simulink model "heatlib_demo"  (R2014b)
settings: Solver=ode1  StartTime=t(1)  StopTime=t(end)  FixedStep=ts  RelTol=1e-3
InitFcn:
  | % Copyright (C) 2014 Kai Kruppa
  | %
  | % This program is free software: you can redistribute it and/or modify it under
  | % the terms of the GNU General Public License as published by the Free Software
  | % Foundation, either version 3 of the License, or (at your option) any later version.
  | %
  | % This program is distributed in the hope that it will be useful, but WITHOUT ANY
  | % WARRANTY; without even the implied warranty of MERCHANTABILITY or
  | % FITNESS FOR A PARTICULAR PURPOSE. See the GNU General Public License for
  | % more details.
  | %
  | % You should have received a copy of the GNU General Public License along with
  | % this program.  If not, see <http://www.gnu.org/licenses/>.
  | 
  | % Kompiliere CMEX-Funktion falls notwendig
  | if exist('storage_tank','file') ~= 3
  |     mex storage_tank.c;
  | end
  | 
  | % Simulationseingang für Modell
  | ts     = 1;
  | N      = 24*60;
  | t      = 60*(0:N-1)';
  | an_aus_BHKW  = ones(N,1);
  | an_aus_Kessel = ones(N,1);
  | dV_ein_Kessel  = [zeros(N/4,1);3/3600*ones(N/2,1);zeros(N/4,1)];
  | dV_ein_BHKW  = [4*ones(N/4,1);1*ones(N/2,1);4*ones(N/4,1)]/3600;
  | an_aus   = [an_aus_Kessel,an_aus_BHKW];
  | dV_ein   = [dV_ein_Kessel,dV_ein_BHKW];
  | dQ_ab   = [50e3*ones(N/4,1);100e3*ones(N/8,1);200e3*ones(N/4,1);150e3*ones(N/8,1);75e3*ones(N/4,1)];
  | dV_V   = [2*ones(N/4,1);3*ones(N/2,1);5*ones(N/4,1)]/3600;
  | T_aussen1 = 20;
  | T_aussen2 = 5;
  | T_aussen = [273+T_aussen1*ones(N/8,1);273+5*ones(3*N/4,1);273+20*ones(N/8,1)];
  | simin = [t, an_aus, dV_ein, dQ_ab, dV_V, T_aussen];
  | 
  | 
  | % Parameter Heizkurve
  | Ta1 = 20;
  | Ta2 = 0;
  | Ts1 = 70;
  | Ts2 = 90;
  | 
  | 
  | % Parameter Kessel:
  | V_K1    = 1;
  | Pmin_K1 = 0;
  | Pmax_K1 = 500;
  | k_K1    = 1e2;
  | c    = 4200;
  | rho  = 1000;
  | KesselNotaus = 273+99;
  | NotausZeit   = 1000;
  | T0_K1   = 273+80;
  | Tu_K1 = 273+30;
  | 
  | % Parameter BHKW
  | V_B = 2;
  | Pmin_B = 10;
  | Pmax_B = 350;
  | k_B = 4e3;
  | T0_B = 273+70;
  | Tu_B = 273+30;
  | 
  | % Parameter Rücklaufanhebung
  | Trl_bhkw_min = 273+50;
  | 
  | % Parameter Speicherkette:
  | k_tank  = 4;    % Anzahl der Speichertanks (1 - 10)
  | n_tank  = 40;   % Anzahl der Rechenknoten pro Tank (1 - 100)
  | mode    = 0;    % Zuflussmodus: '0' feste Position, '1' Schichtladung
  | H_sens  = [1.285, 0.289]; % Anschlusshöhe der Temperatursensoren in einem Speicher [m]
  | T_env   = 273+20;    % Umgebungstemperatur [K]
  | V_tank  = 0.772; % Volumen jedes Speichers [m^3]
  | H_tank  = 1.640; % Höhe jedes Speichers [m]
  | H_in    = 1.469; % Anschlusshöhe des Ladezuflusses [m]
  | H_out   = 0.059; % Anschlusshöhe des Ladeabflusses [m]
  | U_loss  = 9.367; % Wärmedurchgangskoeffizient [W/(m^2 K)]
  | k_eff   = 10.000; % Effektive vertikale Wärmeleitfähigkeit [W/(m K)]
  | T0_mess = linspace(273+50,273+40,length(H_sens)*k_tank);
  |                   % Anfangstemperaturen der Sensoren in allen Speichern [°C]
  | 
  | % Parameter Verbraucher:
  | V_V = 0.1;
  | T0_V  = 273+50;
  | 
  | % Parameter der PID Regler
  | P_bhkw = 0.1;
  | I_bhkw = 0.0001;
  | P_kessel = 1;
  | I_kessel = 1e-5;
StopFcn:
  | % Copyright (C) 2014 Kai Kruppa
  | %
  | % This program is free software: you can redistribute it and/or modify it under
  | % the terms of the GNU General Public License as published by the Free Software
  | % Foundation, either version 3 of the License, or (at your option) any later version.
  | %
  | % This program is distributed in the hope that it will be useful, but WITHOUT ANY
  | % WARRANTY; without even the implied warranty of MERCHANTABILITY or
  | % FITNESS FOR A PARTICULAR PURPOSE. See the GNU General Public License for
  | % more details.
  | %
  | % You should have received a copy of the GNU General Public License along with
  | % this program.  If not, see <http://www.gnu.org/licenses/>.
  | 
  | Tvl_K  = Y(:,1);
  | Trl_K  = Y(:,2);
  | Tvl_V  = Y(:,3);
  | Trl_V  = Y(:,4);
  | T_mess = Y(:,4+(1:length(H_sens)*k_tank));
  | dV_bhkw_vl = Y(:,4+length(H_sens)*k_tank+1);
  | dV_kessel = Y(:,4+length(H_sens)*k_tank+2);
  | mod_bhkw = Y(:,5+length(H_sens)*k_tank+2);
  | mod_kessel = Y(:,6+length(H_sens)*k_tank+2);
  | dV_verb = Y(:,7+length(H_sens)*k_tank+2);
  | T_misch = Y(:,8+length(H_sens)*k_tank+2);
  | 
  | % Heizkurve
  | Ta_min = -10;
  | Ta_max = 30;
  | a = (Ts1 - Ts2)/(Ta1 - Ta2);
  | b = Ts1 - Ta1*a;
  | Ta_plot = [Ta_min:1:Ta_max]';
  | Ts_plot = [Ts2*ones(Ta2-Ta_min,1); a*[Ta2:1:Ta1]'+b; Ts1*ones(Ta_max-Ta1,1)];
  | 
  | figure(1);
  | subplot(4,2,1);
  |     stairs(t/3600,T_aussen-273,'b');
  |     title('Aussentemperatur');
  |     legend('T_{aussen}','Location','SouthEast');
  |     xlabel('Zeit [h]');
  |     ylabel('Temperatur [°C]');
  |     xlim([0 24]);
  |     ylim([0 22]);
  | subplot(4,2,2);
  |     plot(Ta_plot,Ts_plot,'b'); hold on;
  |     plot(T_aussen1, a*T_aussen1+b,'r*');
  |     plot(T_aussen2, a*T_aussen2+b,'g*');hold off
  |     title('Heizkurve');
  |     legend('T_{soll}','T_{aussen} = 20°C','T_{aussen} = 5°C','Location','SouthEast');
  |     xlabel('T_{aussen} [°C]');
  |     ylabel('T_{soll} [°C]');
  |     ylim([65 95]);
  | subplot(4,2,3);
  |     stairs(tsim/3600,Tvl_K-273,'r'); hold on;
  |     stairs(tsim/3600,Trl_K-273,'b');
  |     stairs(tsim/3600,T_misch-273,'g');
  |     hold off;
  |     title({'Gemeinsame Vorlauf- und Rücklauftemperatur von BHKW und Kessel' 'sowie die angehobene Rücklautemperatur des BHKWs'});
  |     legend('Tvl_{ges}','Trl_{ges}', 'Trl_{BHKW}','Location','SouthEast');
  |     xlabel('Zeit [h]');
  |     ylabel('Temperatur [°C]');
  |     xlim([0 24]);
  |     ylim([35 90]);
  | subplot(4,2,4);
  |     stairs(tsim/3600,Tvl_V-273,'r'); hold on;
  |     stairs(tsim/3600,Trl_V-273,'b'); hold off;
  |     title('Gemeinsame Vorlauf- und Rücklauftemperatur der Last');
  |     legend('Tvl_V','Trl_V','Location','SouthEast');
  |     xlabel('Zeit [h]');
  |     ylabel('Temperatur [°C]');
  |     xlim([0 24]);
  |     ylim([25 90]);
  | subplot(4,2,5);
  |     stairs(tsim/3600,T_mess-273,'b');
  |     legend('T_{speicher}','Location','South');
  |     title('Sensortemperaturen in der Speicherkette');
  |     xlabel('Zeit [h]');
  |     ylabel('Temperatur [°C]');
  |     xlim([0 24]);
  |     ylim([35 90]);
  | subplot(4,2,6);
  |     stairs(tsim/3600,mod_kessel,'r'); hold on;
  |     stairs(tsim/3600,mod_bhkw,'b'); hold off;
  |     legend('mod_{Kessel}','mod_{BHKW}','Location','East');
  |     title('Modulationssignale von BHKW und Kessel');
  |     xlabel('Zeit [h]');
  |     ylabel('Modulation');
  |     xlim([0 24]);
  | subplot(4,2,7);
  |     stairs(tsim/3600,(dV_kessel+dV_bhkw_vl-dV_verb)*3600,'b'); hold on;
  |     stairs(t/3600,zeros(N,1),'k:'); hold off;
  |     legend('dV_{speicher}','Location','NorthEast');
  |     title('Volumenstrom im Speicher (positv = laden)');
  |     xlabel('Zeit [h]');
  |     ylabel('Volumenstrom [m^3/h]');
  |     xlim([0 24]);
  | subplot(4,2,8);
  |     stairs(t/3600,dQ_ab/1000,'r');
  |     legend('dQ_{ab}','Location','NorthEast');
  |     title('Abgegebene Leistung in der Last');
  |     xlabel('Zeit [h]');
  |     ylabel('Leistung [kW]');
  |     xlim([0 24]);
  | set(gcf,'Position',[100   100   900   750])
libraries: MatlabHeatLib x7, simulink x2
settings Model: Creator=Kai Kruppa  LastModifiedBy=kathrin
settings SolverCC: AlgebraicLoopSolver=LineSearch
settings DataIOCC: ExternalInput=simin  LimitDataPoints=off  LoadExternalInput=on  SignalLoggingSaveFormat=ModelDataLogs  TimeSaveName=tsim  OutputSaveName=Y
settings OptimizationCC: ExpressionDepthLimit=2147483647
settings DebuggingCC: UnderspecifiedInitializationDetection=Classic  MergeDetectMultiDrivingBlocksExec=none  FcnCallInpInsideContextMsg=EnableAllAsWarning  FrameProcessingCompatibilityMsg=error  StateNameClashWarn=warning

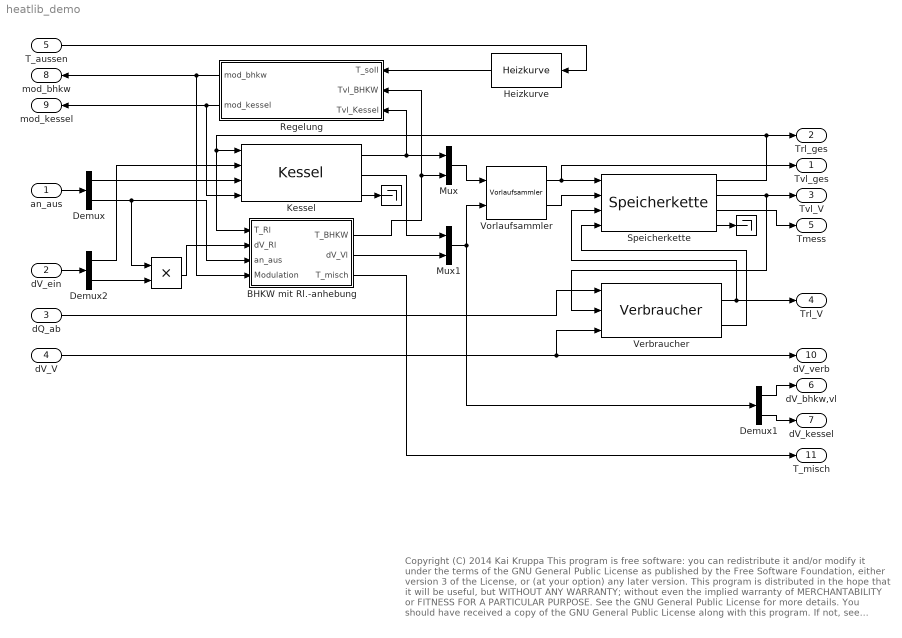
== system heatlib_demo ==
  note: Copyright (C) 2014 Kai Kruppa
      |
      |     This program is free software: you can redistribute it and/or modify it under the terms of the GNU General Public License
      | as published by the Free Software Foundation, either version 3 of the License, or (at your option) any later version.
      |
      | This program is distributed in the hope that it will be useful, but WITHOUT ANY WARRANTY;
      | without even the implied warranty of MERCHANTABILITY or FITNESS FOR A PARTICULAR PURPOSE.
      | See the GNU General Public License for more details.
      |
      |     You should have received a copy of the GNU General Public License along with this program.  If not, see <http://www.gnu.org/licenses/>.
  an_aus : Inport
  dV_ein : Inport  Port=2
  dQ_ab : Inport  Port=3
  dV_V : Inport  Port=4
  T_aussen : Inport  Port=5
  " " : Terminator
  "  " : Terminator
  "    " : Product  RndMeth=Zero
  BHKW mit Rl.-anhebung : Subsystem
  Demux : Demux  Outputs=2
  Demux1 : Demux  Outputs=2
  Demux2 : Demux  Outputs=2
  Heizkurve : MatlabHeatLib/Heizkurve  Ta1c=Ta1  Ta2c=Ta2  Ts1c=Ts1  Ts2c=Ts2
  Kessel : MatlabHeatLib/Kessel  V_Kessel=V_K1  P_min=Pmin_K1  P_max=Pmax_K1  k_Kessel=k_K1  c=c  rho=rho  notaustemp=KesselNotaus  notauszeit=NotausZeit  KesselInit=T0_K1  T_Umgebung=Tu_K1
  Mux : Mux  Inputs=2
  Mux1 : Mux  Inputs=2
  Regelung : Subsystem
  Speicherkette : MatlabHeatLib/Speicherkette  k=k_tank  n=n_tank  mode=mode  Tinit=T0_mess  Hsensors=H_sens  Tenv=T_env  Vtank=V_tank  Htank=H_tank  Hin=H_in  Hout=H_out  U=U_loss  keff=k_eff
  Verbraucher : MatlabHeatLib/Verbraucher  V_Ver=V_V  c=c  rho=rho  InitTempVerbr=T0_V
  Vorlaufsammler : MatlabHeatLib/Vorlaufsammler
  Tvl_ges : Outport
  Trl_ges : Outport  Port=2
  Tvl_V : Outport  Port=3
  Trl_V : Outport  Port=4
  Tmess : Outport  Port=5
  dV_bhkw,vl : Outport  Port=6
  dV_kessel : Outport  Port=7
  mod_bhkw : Outport  Port=8
  mod_kessel : Outport  Port=9
  dV_verb : Outport  Port=10
  T_misch : Outport  Port=11
  wires:
  Verbraucher/1 -> Trl_V/1, Speicherkette/3
  Speicherkette/2 -> Tvl_V/1, Verbraucher/2
  an_aus/1 -> Demux/1
  dV_ein/1 -> Demux2/1
  Demux/2 -> "    "/1, BHKW mit Rl.-anhebung/3(an_aus)
  Kessel/1 -> Mux/1, Regelung/3(Tvl_Kessel)
  Kessel/2 -> Mux1/1
  Mux/1 -> Vorlaufsammler/1
  Mux1/1 -> Vorlaufsammler/2, Demux1/1
  Vorlaufsammler/1 -> Tvl_ges/1, Speicherkette/1
  Vorlaufsammler/2 -> Speicherkette/2
  Speicherkette/1 -> Kessel/1, BHKW mit Rl.-anhebung/1(T_Rl), Trl_ges/1
  dQ_ab/1 -> Verbraucher/1
  dV_V/1 -> dV_verb/1, Verbraucher/3
  Speicherkette/3 -> Tmess/1
  BHKW mit Rl.-anhebung/2(dV_Vl) -> Mux1/2
  Demux2/2 -> "    "/2
  "    "/1 -> BHKW mit Rl.-anhebung/2(dV_Rl)
  BHKW mit Rl.-anhebung/3(T_misch) -> T_misch/1
  BHKW mit Rl.-anhebung/1(T_BHKW) -> Mux/2, Regelung/2(Tvl_BHKW)
  Demux2/1 -> Kessel/2
  Demux/1 -> Kessel/3
  Kessel/3 -> " "/1
  Speicherkette/4 -> "  "/1
  Regelung/2(mod_kessel) -> Kessel/4, mod_kessel/1
  Regelung/1(mod_bhkw) -> BHKW mit Rl.-anhebung/4(Modulation), mod_bhkw/1
  Verbraucher/2 -> Speicherkette/4
  Demux1/1 -> dV_bhkw,vl/1
  Demux1/2 -> dV_kessel/1
  Heizkurve/1 -> Regelung/1(T_soll)
  T_aussen/1 -> Heizkurve/1

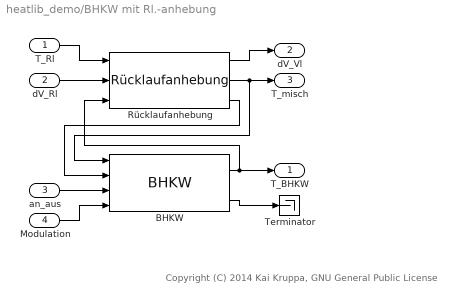
== system heatlib_demo/BHKW mit Rl.-anhebung ==
  note: Copyright (C) 2014 Kai Kruppa, GNU General Public License
  T_Rl : Inport
  dV_Rl : Inport  Port=2
  an_aus : Inport  Port=3
  Modulation : Inport  Port=4
  BHKW : MatlabHeatLib/BHKW  V_BHKW=V_B  P_min=Pmin_B  P_max=Pmax_B  k_BHKW=k_B  c=c  rho=rho  BHKWInit=T0_B  T_Umgebung=Tu_B
  Rücklaufanhebung : MatlabHeatLib/Rücklaufanhebung  T_min=Trl_bhkw_min
  Terminator : Terminator
  T_BHKW : Outport
  dV_Vl : Outport  Port=2
  T_misch : Outport  Port=3
  wires:
  Rücklaufanhebung/3 -> BHKW/2
  BHKW/1 -> T_BHKW/1, Rücklaufanhebung/3
  Rücklaufanhebung/2 -> T_misch/1, BHKW/1
  T_Rl/1 -> Rücklaufanhebung/1
  an_aus/1 -> BHKW/3
  Rücklaufanhebung/1 -> dV_Vl/1
  dV_Rl/1 -> Rücklaufanhebung/2
  Modulation/1 -> BHKW/4
  BHKW/2 -> Terminator/1

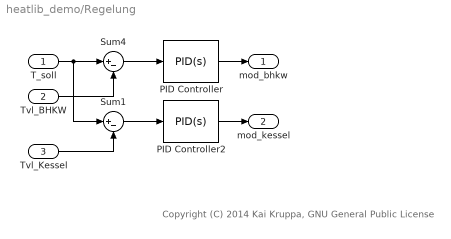
== system heatlib_demo/Regelung ==
  note: Copyright (C) 2014 Kai Kruppa, GNU General Public License
  T_soll : Inport
  Tvl_BHKW : Inport  Port=2
  Tvl_Kessel : Inport  Port=3
  PID Controller : simulink/Continuous/PID Controller  Controller=PID  TimeDomain=Continuous-time  SampleTime=-1  IntegratorMethod=Forward Euler  FilterMethod=Forward Euler  Form=Parallel  UseFilter=on  ControllerParametersSource=internal  P=P_bhkw  I=I_bhkw  D=0  N=100  InitialConditionSource=internal  InitialConditionForIntegrator=0.6  InitialConditionForFilter=0  ExternalReset=none  LimitOutput=on  UpperSaturationLimit=1  LowerSaturationLimit=0  LinearizeAsGain=off  AntiWindupMode=clamping  Kb=1  TrackingMode=off  Kt=1  PParamMin=[]  PParamMax=[]  IParamMin=[]  IParamMax=[]  DParamMin=[]  DParamMax=[]  NParamMin=[]  NParamMax=[]  KbParamMin=[]  KbParamMax=[]  KtParamMin=[]  KtParamMax=[]  POutMin=[]  POutMax=[]  IOutMin=[]  IOutMax=[]  DOutMin=[]  DOutMax=[]  NOutMin=[]  NOutMax=[]  KbOutMin=[]  KbOutMax=[]  KtOutMin=[]  KtOutMax=[]  IntegratorOutMin=[]  IntegratorOutMax=[]  FilterOutMin=[]  FilterOutMax=[]  SumOutMin=[]  SumOutMax=[]  SumI1OutMin=[]  SumI1OutMax=[]  SumI2OutMin=[]  SumI2OutMax=[]  SumI3OutMin=[]  SumI3OutMax=[]  SumDOutMin=[]  SumDOutMax=[]  SaturationOutMin=[]  SaturationOutMax=[]  IntegratorContinuousStateAttributes=''  IntegratorStateMustResolveToSignalObject=off  IntegratorRTWStateStorageClass=Auto  FilterContinuousStateAttributes=''  FilterStateMustResolveToSignalObject=off  FilterRTWStateStorageClass=Auto  DifferentiatorICPrevScaledInput=0  DifferentiatorOutMin=[]  DifferentiatorOutMax=[]
  PID Controller2 : simulink/Continuous/PID Controller  Controller=PID  TimeDomain=Continuous-time  SampleTime=-1  IntegratorMethod=Forward Euler  FilterMethod=Forward Euler  Form=Parallel  UseFilter=on  ControllerParametersSource=internal  P=P_kessel  I=I_kessel  D=0  N=100  InitialConditionSource=internal  InitialConditionForIntegrator=0  InitialConditionForFilter=0  ExternalReset=none  LimitOutput=on  UpperSaturationLimit=1  LowerSaturationLimit=0  LinearizeAsGain=off  AntiWindupMode=clamping  Kb=1  TrackingMode=off  Kt=1  PParamMin=[]  PParamMax=[]  IParamMin=[]  IParamMax=[]  DParamMin=[]  DParamMax=[]  NParamMin=[]  NParamMax=[]  KbParamMin=[]  KbParamMax=[]  KtParamMin=[]  KtParamMax=[]  POutMin=[]  POutMax=[]  IOutMin=[]  IOutMax=[]  DOutMin=[]  DOutMax=[]  NOutMin=[]  NOutMax=[]  KbOutMin=[]  KbOutMax=[]  KtOutMin=[]  KtOutMax=[]  IntegratorOutMin=[]  IntegratorOutMax=[]  FilterOutMin=[]  FilterOutMax=[]  SumOutMin=[]  SumOutMax=[]  SumI1OutMin=[]  SumI1OutMax=[]  SumI2OutMin=[]  SumI2OutMax=[]  SumI3OutMin=[]  SumI3OutMax=[]  SumDOutMin=[]  SumDOutMax=[]  SaturationOutMin=[]  SaturationOutMax=[]  IntegratorContinuousStateAttributes=''  IntegratorStateMustResolveToSignalObject=off  IntegratorRTWStateStorageClass=Auto  FilterContinuousStateAttributes=''  FilterStateMustResolveToSignalObject=off  FilterRTWStateStorageClass=Auto  DifferentiatorICPrevScaledInput=0  DifferentiatorOutMin=[]  DifferentiatorOutMax=[]
  Sum1 : Sum  Inputs=|+-
  Sum4 : Sum  Inputs=|+-
  mod_bhkw : Outport
  mod_kessel : Outport  Port=2
  wires:
  Sum4/1 -> PID Controller/1
  PID Controller/1 -> mod_bhkw/1
  T_soll/1 -> Sum4/1, Sum1/1
  Tvl_Kessel/1 -> Sum1/2
  Sum1/1 -> PID Controller2/1
  PID Controller2/1 -> mod_kessel/1
  Tvl_BHKW/1 -> Sum4/2
